simulink model "TWR-LQR"  (R2020a)
settings: Solver=VariableStepAuto  StartTime=0.0  StopTime=10  RelTol=1e-3
values from neighbouring files (symbols this model uses):
  A = [0     1 ... (first row only)    [TWR-LQR.m]
  Aobs = A-L*C1    [TWR-LQR.m]
  B = [  0 ... (first row only)    [TWR-LQR.m]
  Bobs = [B L]    [TWR-LQR.m]
  Cobs = C    [TWR-LQR.m]
  Dobs = zeros(2)    [TWR-LQR.m]
undefined symbols (not defined in the file or in its folder): K1
settings Model: Creator=Ali  LastModifiedBy=Ali

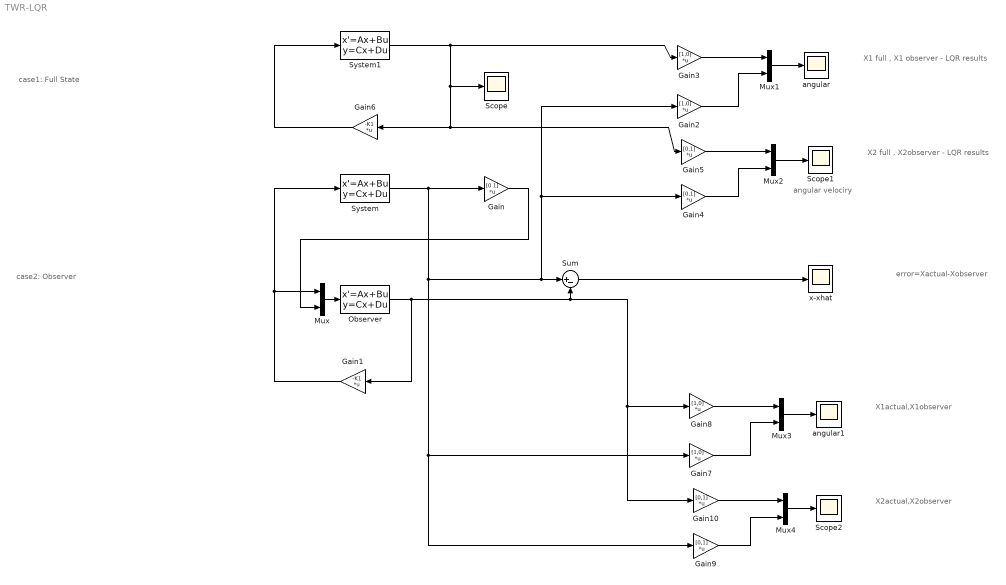
== system TWR-LQR ==
  note: case1: Full State
  note: angular velociry
  note: case2: Observer
  note: X1actual,X1observer
  note: error=Xactual-Xobserver
  note: X1 full , X1 observer - LQR results
  note: X2 full , X2observer - LQR results
  note: X2actual,X2observer
  Gain : Gain  Gain=[0 1]  Multiplication=Matrix(K*u)
  Gain1 : Gain  Gain=-K1  Multiplication=Matrix(K*u)
  Gain{4..5,9..10} (4 alike) : Gain  Gain=[0,1]  Multiplication=Matrix(K*u)
  Gain{2..3,7..8} (4 alike) : Gain  Gain=[1,0]  Multiplication=Matrix(K*u)
  Gain6 : Gain  Gain=-K1  Multiplication=Matrix(K*u)
  Mux{,1..4} (5 alike) : Mux  Inputs=2
  Observer : StateSpace  A=Aobs  B=Bobs  C=Cobs  D=Dobs  InitialCondition=0
  Scope : Scope
  Scope1 : Scope
  Scope2 : Scope
  Sum : Sum  Inputs=|+-
  System : StateSpace  A=A  B=B  C=eye(2)  D=[0;0]  InitialCondition=[20;0]
  System1 : StateSpace  A=A  B=B  C=eye(2)  D=[0;0]  InitialCondition=[20;0]
  angular : Scope
  angular1 : Scope
  x-xhat : Scope
  wires:
  Gain1/1 -> System/1, Mux/1
  Mux/1 -> Observer/1
  Sum/1 -> x-xhat/1
  Gain/1 -> Mux/2
  Gain2/1 -> Mux1/2
  Mux1/1 -> angular/1
  Gain3/1 -> Mux1/1
  Gain6/1 -> System1/1
  System1/1 -> Gain5/1, Gain6/1, Scope/1, Gain3/1
  Gain4/1 -> Mux2/2
  Gain5/1 -> Mux2/1
  Mux2/1 -> Scope1/1
  Gain9/1 -> Mux4/2
  System/1 -> Gain9/1, Gain7/1, Gain4/1, Gain2/1, Sum/1, Gain/1
  Gain10/1 -> Mux4/1
  Gain8/1 -> Mux3/1
  Mux3/1 -> angular1/1
  Gain7/1 -> Mux3/2
  Mux4/1 -> Scope2/1
  Observer/1 -> Gain1/1, Gain10/1, Gain8/1, Sum/2
